simulink model "Boeing787"  (R2013a)
settings: Solver=ode45  SolverMode=SingleTasking  StartTime=0.0  StopTime=10.0  RelTol=1e-3
values from neighbouring files (symbols this model uses):
  FuelBurn = [0 0 0 0 0 0 0 0 0 0 0 0 ... (18249 elements, 1x18249)]    [Benchmark_data1.mat]
undefined symbols (not defined in the file or in its folder): Gearbox_Torque
libraries: PowerFlowLib x27, simulink x5
(part 6 of 6)

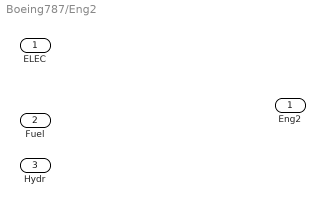
== system Boeing787/Eng2 ==
  ELEC : Inport
  Fuel : Inport  Port=2
  Hydr : Inport  Port=3
  Eng2 : Outport

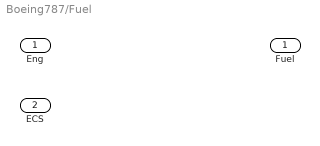
== system Boeing787/Fuel ==
  Eng : Inport
  "ECS " : Inport  Port=2
  Fuel : Outport

== system Boeing787/Hydraulic ==
  Eng : Inport
  "Hydr " : Outport
  wires:
  Eng/1 -> "Hydr "/1

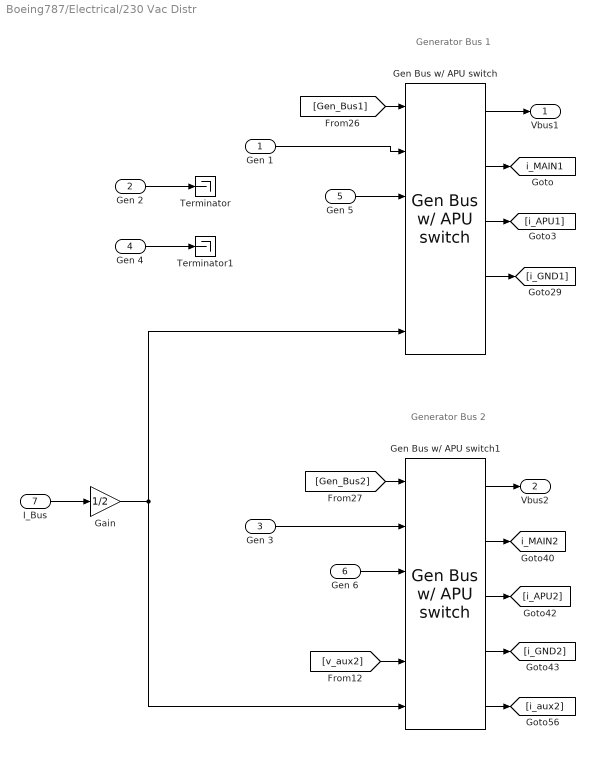
== system Boeing787/Electrical/230 Vac Distr ==
  note: Generator Bus 1
  note: Generator Bus 2
  Gen 1 : Inport
  Gen 2 : Inport  Port=2
  Gen 3 : Inport  Port=3
  Gen 4 : Inport  Port=4
  Gen 5 : Inport  Port=5
  Gen 6 : Inport  Port=6
  I_Bus : Inport  Port=7
  Gain : Gain  Gain=1/2
  Gen Bus w/ APU switch : PowerFlowLib/Energy & Power Systems/Electrical/Systems/Gen Bus w// APU switch  LOWVLIMIT=90  UPVLIMIT=250  bus_st=2
  Gen Bus w/ APU switch1 : PowerFlowLib/Energy & Power Systems/Electrical/Systems/Gen Bus w// APU switch  LOWVLIMIT=90  UPVLIMIT=250  bus_st=2
  Terminator : Terminator
  Terminator1 : Terminator
  Vbus1 : Outport
  Vbus2 : Outport  Port=2
  tag scope: i_MAIN1=global, i_MAIN2=global
  wires:
  Gen Bus w/ APU switch/3 -> [i_APU1]
  Gen Bus w/ APU switch/4 -> [i_GND1]
  [Gen_Bus1] -> Gen Bus w/ APU switch/1
  Gen Bus w/ APU switch/2 -> [i_MAIN1]
  Gen Bus w/ APU switch1/3 -> [i_APU2]
  Gen Bus w/ APU switch1/4 -> [i_GND2]
  Gen Bus w/ APU switch1/2 -> [i_MAIN2]
  [Gen_Bus2] -> Gen Bus w/ APU switch1/1
  [v_aux2] -> Gen Bus w/ APU switch1/5
  Gen Bus w/ APU switch1/5 -> [i_aux2]
  Gen 1/1 -> Gen Bus w/ APU switch/2
  Gen 3/1 -> Gen Bus w/ APU switch1/2
  Gen 5/1 -> Gen Bus w/ APU switch/3
  Gen 6/1 -> Gen Bus w/ APU switch1/3
  Gen Bus w/ APU switch/1 -> Vbus1/1
  Gen Bus w/ APU switch1/1 -> Vbus2/1
  I_Bus/1 -> Gain/1
  Gain/1 -> Gen Bus w/ APU switch/6, Gen Bus w/ APU switch1/6
  Gen 2/1 -> Terminator/1
  Gen 4/1 -> Terminator1/1

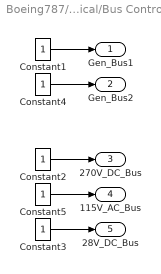
== system Boeing787/Electrical/Bus Controls ==
  Constant{1..5} (5 alike) : Constant
  Gen_Bus1 : Outport
  Gen_Bus2 : Outport  Port=2
  270V_DC_Bus : Outport  Port=3
  115V_AC_Bus : Outport  Port=4
  28V_DC_Bus : Outport  Port=5
  wires:
  Constant3/1 -> 28V_DC_Bus/1
  Constant5/1 -> 115V_AC_Bus/1
  Constant2/1 -> 270V_DC_Bus/1
  Constant4/1 -> Gen_Bus2/1
  Constant1/1 -> Gen_Bus1/1

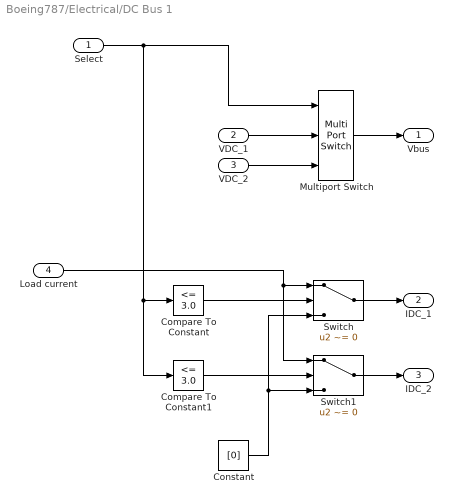
== system Boeing787/Electrical/DC Bus 1 ==
  Select : Inport
  VDC_1 : Inport  Port=2
  VDC_2 : Inport  Port=3
  Load current : Inport  Port=4
  Compare To Constant : simulink/Logic and Bit Operations/Compare To Constant  relop=<=  const=3.0  OutDataTypeStr=boolean
  Compare To Constant1 : simulink/Logic and Bit Operations/Compare To Constant  relop=<=  const=3.0  OutDataTypeStr=boolean
  Constant : Constant  Value=[0]
  Multiport Switch : MultiPortSwitch  Inputs=2
  Switch : Switch  Criteria=u2 ~= 0
  Switch1 : Switch  Criteria=u2 ~= 0
  Vbus : Outport
  IDC_1 : Outport  Port=2
  IDC_2 : Outport  Port=3
  wires:
  Load current/1 -> Switch1/1, Switch/1
  Multiport Switch/1 -> Vbus/1
  VDC_1/1 -> Multiport Switch/2
  VDC_2/1 -> Multiport Switch/3
  Select/1 -> Multiport Switch/1, Compare To Constant/1, Compare To Constant1/1
  Compare To Constant/1 -> Switch/2
  Compare To Constant1/1 -> Switch1/2
  Constant/1 -> Switch/3, Switch1/3
  Switch/1 -> IDC_1/1
  Switch1/1 -> IDC_2/1

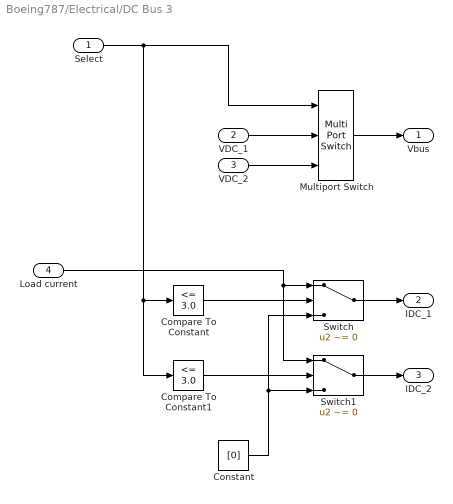
== system Boeing787/Electrical/DC Bus 3 ==
  Select : Inport
  VDC_1 : Inport  Port=2
  VDC_2 : Inport  Port=3
  Load current : Inport  Port=4
  Compare To Constant : simulink/Logic and Bit Operations/Compare To Constant  relop=<=  const=3.0  OutDataTypeStr=boolean
  Compare To Constant1 : simulink/Logic and Bit Operations/Compare To Constant  relop=<=  const=3.0  OutDataTypeStr=boolean
  Constant : Constant  Value=[0]
  Multiport Switch : MultiPortSwitch  Inputs=2
  Switch : Switch  Criteria=u2 ~= 0
  Switch1 : Switch  Criteria=u2 ~= 0
  Vbus : Outport
  IDC_1 : Outport  Port=2
  IDC_2 : Outport  Port=3
  wires:
  Load current/1 -> Switch1/1, Switch/1
  Multiport Switch/1 -> Vbus/1
  VDC_1/1 -> Multiport Switch/2
  VDC_2/1 -> Multiport Switch/3
  Select/1 -> Multiport Switch/1, Compare To Constant/1, Compare To Constant1/1
  Compare To Constant/1 -> Switch/2
  Compare To Constant1/1 -> Switch1/2
  Constant/1 -> Switch/3, Switch1/3
  Switch/1 -> IDC_1/1
  Switch1/1 -> IDC_2/1

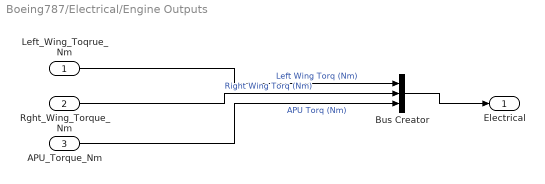
== system Boeing787/Electrical/Engine Outputs ==
  Left_Wing_Toqrue_Nm : Inport
  Rght_Wing_Torque_Nm : Inport  Port=2
  APU_Torque_Nm : Inport  Port=3
  Bus Creator : BusCreator  Inputs=3
  Electrical : Outport
  wires:
  Rght_Wing_Torque_Nm/1 -> Bus Creator/2  "Right Wing Torq (Nm)"
  APU_Torque_Nm/1 -> Bus Creator/3  "APU Torq (Nm)"
  Left_Wing_Toqrue_Nm/1 -> Bus Creator/1  "Left Wing Torq (Nm)"
  Bus Creator/1 -> Electrical/1

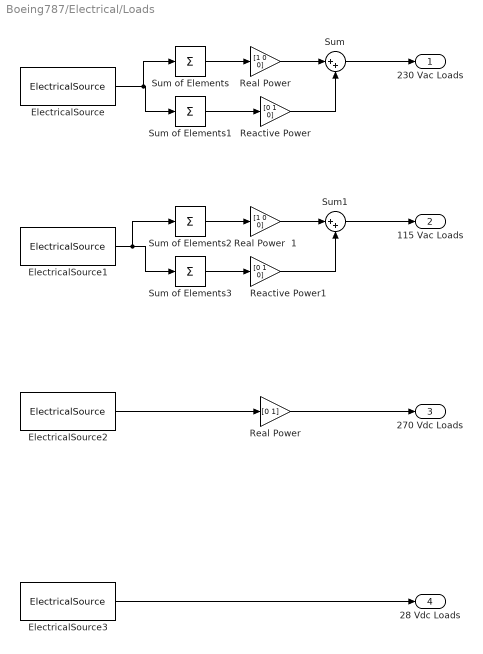
== system Boeing787/Electrical/Loads ==
  ElectricalSource{,1..3} (4 alike) : PowerFlowLib/Support Functions//Tools/ElectricalSource  Tag=Flow  Description=TwoPhase  load_loc=Cockpit  ACDC_load=DC
  Reactive Power : Gain  Gain=[0 1 0]
  Reactive Power1 : Gain  Gain=[0 1 0]
  "Real Power " : Gain  Gain=[0 1]
  "Real Power  " : Gain  Gain=[1 0 0]
  Real Power  1 : Gain  Gain=[1 0 0]
  Sum : Sum  Inputs=|++
  Sum of Elements{,1..3} (4 alike) : Sum  Inputs=+
  Sum1 : Sum  Inputs=|++
  230 Vac Loads : Outport
  115 Vac Loads : Outport  Port=2
  270 Vdc Loads : Outport  Port=3
  28 Vdc Loads : Outport  Port=4
  wires:
  "Real Power  "/1 -> Sum/1
  Reactive Power/1 -> Sum/2
  Sum of Elements/1 -> "Real Power  "/1
  Sum of Elements1/1 -> Reactive Power/1
  Sum/1 -> 230 Vac Loads/1
  ElectricalSource1/1 -> Sum of Elements2/1, Sum of Elements3/1
  Real Power  1/1 -> Sum1/1
  Reactive Power1/1 -> Sum1/2
  Sum of Elements2/1 -> Real Power  1/1
  Sum of Elements3/1 -> Reactive Power1/1
  Sum1/1 -> 115 Vac Loads/1
  "Real Power "/1 -> 270 Vdc Loads/1
  ElectricalSource2/1 -> "Real Power "/1
  ElectricalSource3/1 -> 28 Vdc Loads/1
  ElectricalSource/1 -> Sum of Elements/1, Sum of Elements1/1

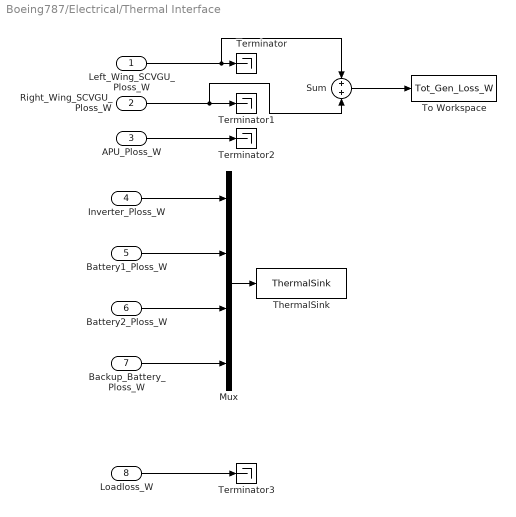
== system Boeing787/Electrical/Thermal Interface ==
  Left_Wing_SCVGU_Ploss_W : Inport
  Right_Wing_SCVGU_Ploss_W : Inport  Port=2
  APU_Ploss_W : Inport  Port=3
  Inverter_Ploss_W : Inport  Port=4
  Battery1_Ploss_W : Inport  Port=5
  Battery2_Ploss_W : Inport  Port=6
  Backup_Battery_Ploss_W : Inport  Port=7
  Loadloss_W : Inport  Port=8
  Mux : Mux
  Sum : Sum
  Terminator{,1..3} (4 alike) : Terminator
  ThermalSink : PowerFlowLib/Support Functions//Tools/ThermalSink  Tag=Flow  Description=TwoPhase  load_loc=Cabin  units=Watts  unq_id=8332
  To Workspace : ToWorkspace  VariableName=Tot_Gen_Loss_W  SampleTime=10  SaveFormat=Structure With Time
  wires:
  Right_Wing_SCVGU_Ploss_W/1 -> Sum/2, Terminator1/1
  APU_Ploss_W/1 -> Terminator2/1
  Mux/1 -> ThermalSink/1
  Inverter_Ploss_W/1 -> Mux/1
  Battery1_Ploss_W/1 -> Mux/2
  Battery2_Ploss_W/1 -> Mux/3
  Backup_Battery_Ploss_W/1 -> Mux/4
  Loadloss_W/1 -> Terminator3/1
  Left_Wing_SCVGU_Ploss_W/1 -> Sum/1, Terminator/1
  Sum/1 -> To Workspace/1

== system Boeing787/Eng1/Unit Conversion 1 ==
  Signal_in : Inport
  conv_fcn : Fcn  Expr=u(1)/1.8
  Converted Signal Out : Outport
  wires:
  conv_fcn/1 -> Converted Signal Out/1
  Signal_in/1 -> conv_fcn/1

== system Boeing787/Eng1/Unit Conversion 4 ==
  Signal_in : Inport
  conv_fcn : Fcn  Expr=u(1)/(1.450377e-1)
  Converted Signal Out : Outport
  wires:
  Signal_in/1 -> conv_fcn/1
  conv_fcn/1 -> Converted Signal Out/1

== system Boeing787/Eng1/Unit Conversion 5 ==
  Signal_in : Inport
  conv_fcn : Fcn  Expr=u(1)*.45359237
  Converted Signal Out : Outport
  wires:
  Signal_in/1 -> conv_fcn/1
  conv_fcn/1 -> Converted Signal Out/1
